simulink model "s_apol1"  (Simulink 4.00)
settings: Solver=ode45  SolverMode=SingleTasking  StartTime=0.0  StopTime=999999  MaxStep=10  RelTol=1e-3  AbsTol=1e-6
values from neighbouring files (symbols this model uses):
  A = [Ap, Bp*Cs; zeros(ns,np), As]    [akalm1.m]    (also in kalm1.m = my_sys1.a; kalm2.m = my_sys1.a; kalm3.m = my_sys1.a; kalm4.m = zeros(6,6))
  B = [Bp; zeros(ns,1)]    [akalm1.m]    (also in kalm1.m = my_sys1.b; kalm2.m = my_sys1.b; kalm3.m = my_sys1.b; kalm4.m = [zeros(3,3); 1/m1, 0, 0; 0, 1/m2, 0; 0, 0, 1/m3])
  C = [Cp, zeros(1,ns)]    [akalm1.m]    (also in kalm1.m = my_sys1.c; kalm2.m = my_sys1.c; kalm3.m = my_sys1.c; kalm4.m = [eye(3,3), zeros(3,3)])
  D = [0]    [akalm1.m]    (also in kalm1.m = my_sys1.d; kalm2.m = my_sys1.d; kalm3.m = my_sys1.d; kalm4.m = zeros(3,3))
  K = lqrd(A, B, Q, R, Ts)    [abeob1.m]    (also in apol1.m = place(A, B, p); kalm3.m = K*0; kalm4.m = K_temp; lqr_2.m = place(A',C',p))
  x0 = [5, 0, 0, 0]    [abeob1.m]    (also in alqr1.m; alqrd1.m; apol1.m; estimate_1.m = [1 2 3])
settings Model: LastModifiedBy=Administrator  SaveTime=off  SaveOutput=off  LimitDataPoints=off  BlockReductionOpt=off

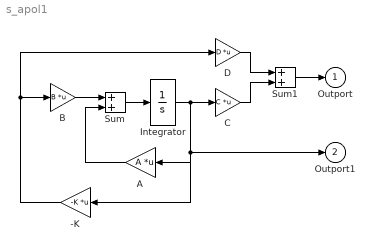
== system s_apol1 ==
  -K : Gain  Orientation=left  Gain=-K  Multiplication=Matrix(K*u)  SaturateOnIntegerOverflow=on
  A : Gain  Orientation=left  Gain=A  Multiplication=Matrix(K*u)  SaturateOnIntegerOverflow=on
  B : Gain  Gain=B  Multiplication=Matrix(K*u)  SaturateOnIntegerOverflow=on
  C : Gain  Gain=C  Multiplication=Matrix(K*u)  SaturateOnIntegerOverflow=on
  D : Gain  Gain=D  Multiplication=Matrix(K*u)  SaturateOnIntegerOverflow=on
  Integrator : Integrator  ExternalReset=none  InitialConditionSource=internal  InitialCondition=x0  LimitOutput=off  UpperSaturationLimit=inf  LowerSaturationLimit=-inf  ShowSaturationPort=off  ShowStatePort=off  AbsoluteTolerance=auto
  Sum : Sum  Inputs=++  SaturateOnIntegerOverflow=on
  Sum1 : Sum  Inputs=++  SaturateOnIntegerOverflow=on
  Outport : Outport  Port=1
  Outport1 : Outport  Port=2
  wires:
  -K/1 -> B/1, D/1
  Sum1/1 -> Outport/1
  C/1 -> Sum1/2
  D/1 -> Sum1/1
  B/1 -> Sum/1
  A/1 -> Sum/2
  Sum/1 -> Integrator/1
  Integrator/1 -> -K/1, C/1, A/1, Outport1/1
